simulink model "main"  (R2022b)
settings: Solver=VariableStepAuto  StartTime=0.0  StopTime=10  RelTol=1e-6
InitFcn:
  | test
values from neighbouring files (symbols this model uses):
  A_cc = [0 1 0 ... (first row only)    [test.m]
  A_esp = [-16.95,  -2.365 ... (first row only)    [test.m]
  A_sc = [3.957e-14  1  1.351e-14   1.193e-16 ... (first row only)    [test.m]
  A_ttc = [0,1;0,0]    [test.m]
  B_cc = [0; 0; 2.4767]    [test.m]
  B_esp = [8.478 ... (first row only)    [test.m]
  B_sc = [9.628e-15; 80; 20; -1120]    [test.m]
  B_ttc = [0;1]    [test.m]
  C_cc1 = eye(size(A_cc,1))    [test.m]
  C_esp1 = eye(size(A_esp,1))    [test.m]
  C_sc1 = eye(size(A_sc,1))    [test.m]
  C_ttc1 = eye(size(A_ttc,1))    [test.m]
  D_cc1 = zeros(size(A_cc,1),size(B_cc,2))    [test.m]
  D_esp1 = zeros(size(A_esp,1),size(B_esp,2))    [test.m]
  D_sc1 = zeros(size(A_sc,1),size(B_sc,2))    [test.m]
  D_ttc1 = zeros(size(A_ttc,1),size(B_ttc,2))    [test.m]
undefined symbols (not defined in the file or in its folder): sharedmem
libraries: truetime x2
settings Model: Creator=anton  LastModifiedBy=sunan
settings SolverCC: AlgebraicLoopSolver=TrustRegion
settings DataIOCC: ReturnWorkspaceOutputs=off
settings DebuggingCC: UnconnectedInputMsg=warning  UnconnectedOutputMsg=warning  UnconnectedLineMsg=warning  SFMachineParentedDataDiag=warning  ArithmeticOperatorsInVariantConditions=warning
settings ModelReferenceCC: EnableRefExpFcnMdlSchedulingChecks=on
settings SFSimCC: SimUseLocalCustomCode=off  CustomCodeUndefinedFunction=UseInterfaceOnly
settings RTWCC: RTWUseLocalCustomCode=off  DLArmComputeVersion=19.05
settings CodeAppCC: StateflowObjectComments=on

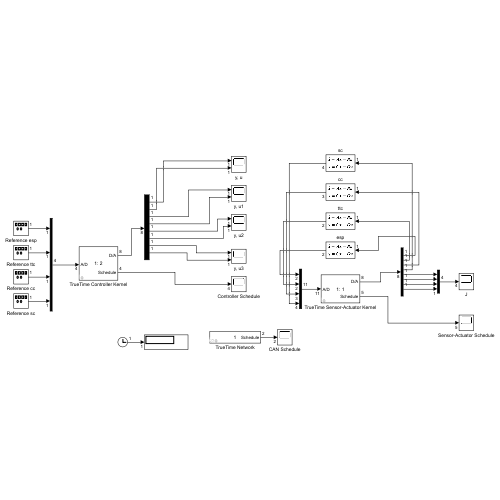
[thumbnail: Simulink's stored preview of the top-level diagram]
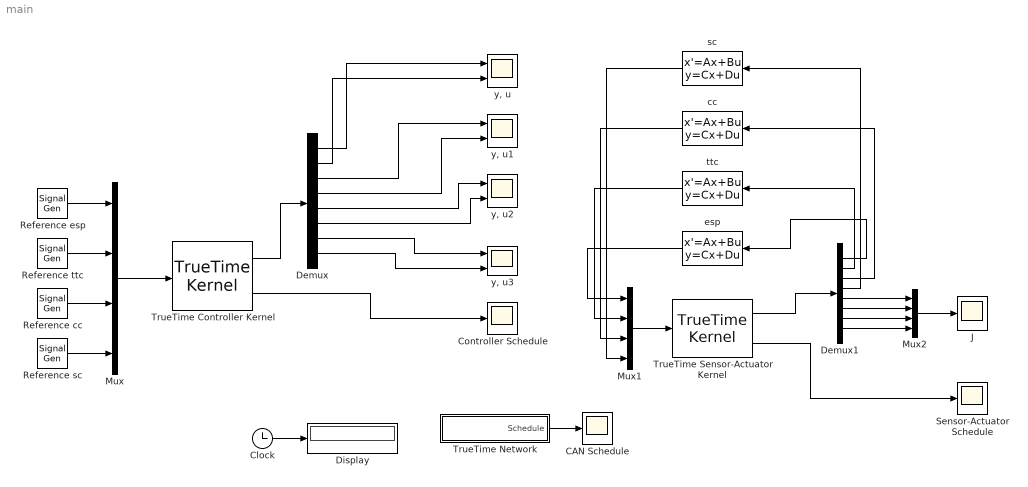
== system main ==
  CAN Schedule : Scope
  Clock : Clock
  Controller Schedule : Scope
  Demux : Demux  Outputs=8
  Demux1 : Demux  Outputs=8
  Display : Display
  J : Scope
  Mux : Mux
  Mux1 : Mux
  Mux2 : Mux
  Reference cc : SignalGenerator  WaveForm=square  Amplitude=-1  Frequency=0.02
  Reference esp : SignalGenerator  WaveForm=square  Amplitude=-10  Frequency=0.02
  Reference sc : SignalGenerator  WaveForm=square  Amplitude=-1  Frequency=0.02
  Reference ttc : SignalGenerator  WaveForm=square  Amplitude=-1  Frequency=0.02
  Sensor-Actuator Schedule : Scope
  TrueTime Controller Kernel : truetime/TrueTime Kernel  sfun=control_sched_init  args=Systems  ninputsoutputs=[4 8]  ntriggers=0  trigtype=falling  nwnodenbr=2  clockoffsetdrift=[0 0]  schedoutput=on  battery=off  poweroutput=off  label=1: 2
  TrueTime Network : Subsystem  AncestorBlock=truetime/TrueTime Network  mask(Real-Time Network){nwtype=CSMA/AMP (CAN), nwnbr=1, nnodes=2, rate=500000, minsize=64, lossprob=0, seed=0, bandwidths=[0.5 0.5], slotsize=512, schedule=[1 1 2], memsize=80000, buftype=Common buffer, overflow=Retransmit, dynSchedule=0, miniSlotSize=0, NIT=0, QSortMode=FIFO, sync=0, irtSchedule=0, nrtLength=0, nodeGraph=0, scheduleoutput=on}
      mask prompts: nwtype "Network type:"; nwnbr "Network number:"; nnodes "Number of nodes:"; rate "Data rate (bits/s):"; minsize "Minimum frame size (bits):"; lossprob "Loss probability (0-1):"; seed "Initial seed:"; bandwidths "Bandwidth allocations:"; slotsize "Slotsize (bits):"; schedule "Static schedule:"; memsize "Total switch memory (bits):"; buftype "Switch buffer type:"; overflow "Switch overflow behavior:"; dynSchedule "Dynamic Schedule:"; miniSlotSize "Mini slot size (bits):"; NIT "Network idle time (bits):"; QSortMode "Input Queue Sorted by:"; sync "Synchronization length (bits):"; irtSchedule "IRT Schedule [msgID from to start arrival]:"; nrtLength "RT Class 1/NRT length (bits):"; nodeGraph "Node connection graph (nbrOfnodes x nbrOfNodes):"; scheduleoutput "Show Schedule output port:"
      mask init:
      | ttnetwork_callback(gcb,nwnbr,nnodes,scheduleoutput)
      mask TypeOptions nwtype: CSMA/CD (Ethernet) | CSMA/AMP (CAN) | Round Robin | FDMA | TDMA | Switched Ethernet | FlexRay | PROFINET | NCM
      mask Callback nwtype: ttnetwork_callback
      mask TypeOptions buftype: Common buffer | Symmetric output buffers
      mask TypeOptions overflow: Retransmit | Drop
      mask TypeOptions QSortMode: FIFO | Priority
      mask Display: disp(nwnbr)
  TrueTime Sensor-Actuator Kernel : truetime/TrueTime Kernel  sfun=sensact_sched_init  args=Systems  ninputsoutputs=[4 8]  ntriggers=0  trigtype=falling  nwnodenbr=1  clockoffsetdrift=[0 0]  schedoutput=on  battery=off  poweroutput=off  label=1: 1
  cc : StateSpace  A=A_cc  B=B_cc  C=C_cc1  D=D_cc1  InitialCondition=sharedmem.x0{3}
  esp : StateSpace  A=A_esp  B=B_esp  C=C_esp1  D=D_esp1  InitialCondition=sharedmem.x0{1}
  sc : StateSpace  A=A_sc  B=B_sc  C=C_sc1  D=D_sc1  InitialCondition=sharedmem.x0{4}
  ttc : StateSpace  A=A_ttc  B=B_ttc  C=C_ttc1  D=D_ttc1  InitialCondition=sharedmem.x0{2}
  y, u{,1..3} (4 alike) : Scope  NumInputPorts=2
  wires:
  TrueTime Controller Kernel/2 -> Controller Schedule/1
  Demux/2 -> "y, u"/2
  TrueTime Controller Kernel/1 -> Demux/1
  Demux/1 -> "y, u"/1
  TrueTime Network/1(Schedule) -> CAN Schedule/1
  TrueTime Sensor-Actuator Kernel/1 -> Demux1/1
  TrueTime Sensor-Actuator Kernel/2 -> Sensor-Actuator Schedule/1
  Mux/1 -> TrueTime Controller Kernel/1
  Reference esp/1 -> Mux/1
  Reference ttc/1 -> Mux/2
  Reference sc/1 -> Mux/4
  Reference cc/1 -> Mux/3
  Clock/1 -> Display/1
  Mux1/1 -> TrueTime Sensor-Actuator Kernel/1
  Demux1/1 -> esp/1
  Demux1/2 -> ttc/1
  Demux1/3 -> cc/1
  Demux1/4 -> sc/1
  Demux1/5 -> Mux2/1
  Demux1/6 -> Mux2/2
  Demux1/7 -> Mux2/3
  Demux1/8 -> Mux2/4
  Mux2/1 -> J/1
  esp/1 -> Mux1/1
  ttc/1 -> Mux1/2
  cc/1 -> Mux1/3
  sc/1 -> Mux1/4
  Demux/3 -> "y, u1"/1
  Demux/4 -> "y, u1"/2
  Demux/5 -> "y, u2"/1
  Demux/6 -> "y, u2"/2
  Demux/7 -> "y, u3"/1
  Demux/8 -> "y, u3"/2

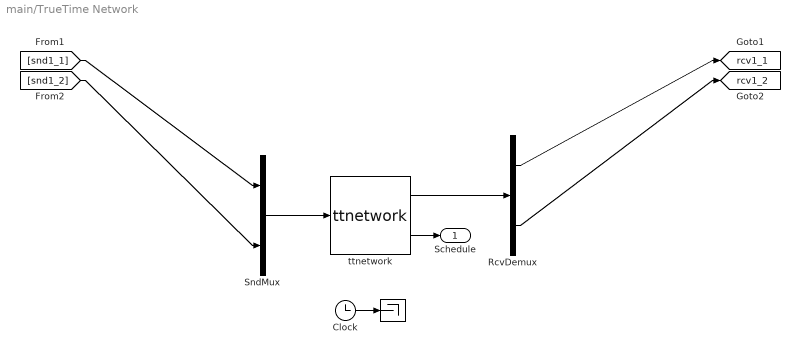
== system main/TrueTime Network ==
  " " : Terminator
  Clock : Clock
  RcvDemux : Demux  Outputs=2
      settings: DisplayOption=none
  SndMux : Mux  Inputs=2
  ttnetwork : S-Function  FunctionName=ttnetwork  Parameters=nwtype,nwnbr,nnodes,rate,minsize,lossprob,bandwidths,slotsize,schedule,memsize,buftype,overflow,seed,dynSchedule,miniSlotSize,NIT,QSortMode,sync,irtSchedule,nrtLength,nodeGraph  SFunctionDeploymentMode=off  EnableBusSupport=off
  Schedule : Outport
  tag scope: rcv1_1=global, rcv1_2=global
  wires:
  Clock/1 -> " "/1
  SndMux/1 -> ttnetwork/1
  ttnetwork/1 -> RcvDemux/1
  ttnetwork/2 -> Schedule/1
  [snd1_1] -> SndMux/1
  [snd1_2] -> SndMux/2
  RcvDemux/1 -> [rcv1_1]
  RcvDemux/2 -> [rcv1_2]
